simulink model "SailingYachtModel"  (R2017a)
settings: Solver=ode3  StartTime=0.0  StopTime=1800  FixedStep=0.4  RelTol=1e-3
settings Model: Creator=Administrator  LastModifiedBy=davi
settings DataIOCC: LimitDataPoints=on  SaveFormat=Array  SignalLoggingSaveFormat=ModelDataLogs
settings OptimizationCC: BlockReduction=off  BooleanDataType=off  LifeSpan=inf
settings DebuggingCC: SaveWithParameterizedLinksMsg=none  UnderspecifiedInitializationDetection=Classic  MergeDetectMultiDrivingBlocksExec=none  SignalResolutionControl=TryResolveAllWithWarning  MultiTaskDSMMsg=warning  MultiTaskCondExecSysMsg=none  StateNameClashWarn=warning  SFUnexpectedBacktrackingDiag=warning  SFNoUnconditionalDefaultTransitionDiag=warning  SFExecutionAtInitializationDiag=none
settings HardwareCC: ProdBitPerPointer=32  ProdBitPerSizeT=32  ProdBitPerPtrDiffT=32  ProdLargestAtomicFloat=None  ProdIntDivRoundTo=Undefined  ProdEndianess=Unspecified  ProdWordSize=32  ProdHWDeviceType=32-bit Generic  TargetUnknown=on
settings ModelReferenceCC: PropagateSignalLabelsOutOfModel=off
settings GRTTargetCC: TargetLangStandard=C89/C90 (ANSI)  GeneratePreprocessorConditionals=Disable all
settings ConfigComp: CovMetricSettings=dw  CovHtmlReporting=on  CovSaveCumulativeToWorkspaceVar=on  CovSaveSingleToWorkspaceVar=on  CovExternalEMLEnable=off

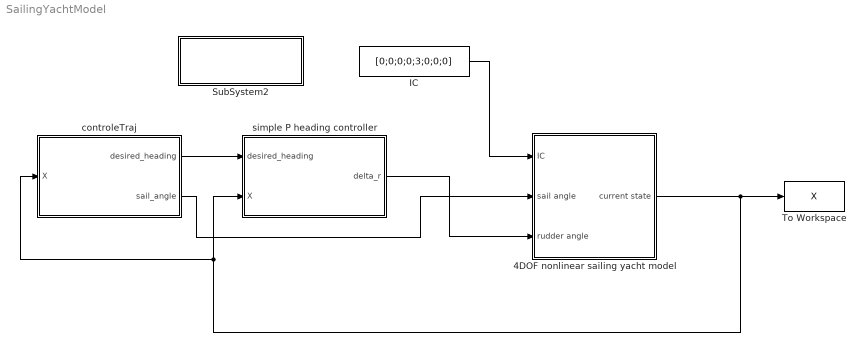
== system SailingYachtModel ==
  4DOF nonlinear sailing yacht model : Subsystem
  IC : Constant  Value=[0;0;0;0;3;0;0;0]
  SubSystem2 : Subsystem  InitFcn=|
      | global par                                                                      
      | par.dist_lateral = 0;                                                           
      | par.contador_teste = 1;                                                         
      | par.overshoot = 0;                                                              
      | par.tempopico = 0;                                                              
      | par.temposub = 0;                                                               
      | par.flagtemposub = true;                                                        
      | par.flagAcomod = false;                                                         
      | par.tempoDeAcomod = 0;                                                          
      | par.spvec = 0;                                                                  
      | par.spveccont = 1;                                                              
      | par.lastDistanciaAlvo = 0;                                                      
      | par.flag = 0;                                                                   
      | par.contador_bug = 0;                                                           
      | par.psi = 0;                                                                    
      | par.velocidade = 0;                                                             
      | par.contVel = 1;                                                                
      | par.Ianterior = 0;                                                              
      | par.distanciaAlvo = 999999999                                                   
      | w1 = [200;0];
      | w2 = [100;100];
      | w3 = [0;0];                                                                                                     
      | par.waypoints = [w1];                                                     
      | par.waypointId = 1;                                                             
      | par.nextLocation = [0;0];                                                       
      | par.waypointBId = 1;                                                            
      | par.isBordejando = false;                                                       
      | par.i = 1;                                                                      
      | par.pontos_bordejar = eye(2,1);                                                 
      | par.controle = 0;                                                               
      | par.lastlastLocation = eye(2,1);                                                
      | par.taxa_dist = 0.3;                                                            
      | par.angulo_bordejo = 40;                                                        
      | par.m = 25900;                         % (kg),mass of the vehicle               
      | par.Ixx = 133690;                                                               
      | par.Izz = 24760;                                                                
      | par.Ixz = 2180;                        % moment of inertia                      
      | par.a11 = 970;                                                                  
      | par.a22 = 17430;                                                                
      | par.a44 = 106500;                                                               
      | par.a66 = 101650;                                                               
      | par.a24 = -13160;                                                               
      | par.a26 = -6190;                                                                
      | par.a46 = 4730;                        % (kg),added mass coef.                  
      |                                                                                 
      | par.vt = 10;                           % the norm of wind velocity              
      |                                                                                 
      | par.rho_a = 1.2;                       % (kg/m^3), air density                  
      | par.As = 170;                          % (m^2), sail area                       
      | par.h0 = 0.0005;                       % (m), roughness height                  
      | par.h1 = 11.58;                        % (m), reference height                  
      | par.z_s = -11.58;                      % (m), (x,y,z) is the CoE                
      | par.xs = 0;                                                                     
      | par.ys = 0;                                                                     
      | par.zs = -11.58;                       % (m), (x,y,z) is the CoE                
      | par.Xce = 0.6;                         % (m), distance along the mast to the CoE
      | par.Xm = 0.3;                          % (m), x-coordinate of the mast          
      |                                                                                 
      | par.rho_w = 1025;                      % (kg/m^3), water density                
      | par.Ar = 1.17;                         % (m^2), rudder area                     
      | par.d_r = 1.9;                         % rudder draft                           
      | par.zeta_r = 0.8;                      % rudder efficiency                      
      | par.x_r = -8.2;                                                                 
      | par.z_r = -0.78;                       % (m), (x,y,z) is the CoE                
      | par.xr = -8.2;                                                                  
      | par.yr = 0;                                                                     
      | par.zr = -0.78;                        % (m), (x,y,z) is the CoE                
      |                                                                                 
      | par.Ak = 8.7;                          % (m^2), keel area                       
      | par.d_k = 2.49;                        % keel draft                             
      | par.zeta_k = 0.7;                      % keel efficiency                        
      | par.x_k = 0;                                                                    
      | par.z_k = -0.58;                       % (m), (x,y,z) is the CoE                
      | par.xk = 0;                                                                     
      | par.yk = 0;                                                                     
      | par.zk = -0.58;                        % (m), (x,y,z) is the CoE                
      |                                                                                 
      | par.x_h = 0;                                                                    
      | par.z_h = -1.18;                       % (m), (x,y,z) is the CoE                
      | par.xh = 0;                                                                     
      | par.yh = 0;                                                                     
      | par.zh = -1.18;                        % (m), (x,y,z) is the CoE                
      |                                                                                 
      | par.w_c = 60000;                       % (N), crew weight 20000                 
      | par.x_c = -8;                          % (m), crew position                     
      | par.y_bm = 3.6;                        % (m), yacht beam                        
      |                                                                                 
      | par.a = -5.89;                                                                  
      | par.b = 8160;                                                                   
      | par.c = 120000;                                                                 
      | par.d = 50000;
      mask Display: disp('Parameter Initialization')
  To Workspace : ToWorkspace  VariableName=X  SaveFormat=Structure With Time  SampleTime=-1
  controleTraj : Subsystem
  simple P heading controller : Subsystem
  wires:
  controleTraj/1(desired_heading) -> simple P heading controller/1(desired_heading)
  4DOF nonlinear sailing yacht model/1(current state) -> controleTraj/1(X), simple P heading controller/2(X), To Workspace/1
  IC/1 -> 4DOF nonlinear sailing yacht model/1(IC)
  controleTraj/2(sail_angle) -> 4DOF nonlinear sailing yacht model/2(sail angle)
  simple P heading controller/1(delta_r) -> 4DOF nonlinear sailing yacht model/3(rudder angle)

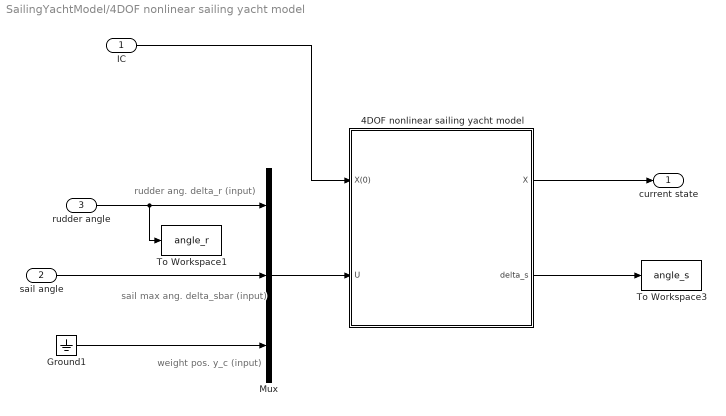
== system SailingYachtModel/4DOF nonlinear sailing yacht model ==
  note: weight pos. y_c (input)
  note: rudder ang. delta_r (input)
  note: sail max ang. delta_sbar (input)
  IC : Inport
  sail angle : Inport  Port=2
  rudder angle : Inport  Port=3
  4DOF nonlinear sailing yacht model : Subsystem
  Ground1 : Ground
  Mux : Mux  Inputs=3
  To Workspace1 : ToWorkspace  VariableName=angle_r  SaveFormat=Structure With Time  SampleTime=-1
  To Workspace3 : ToWorkspace  VariableName=angle_s  SaveFormat=Structure With Time  SampleTime=-1
  current state : Outport
  wires:
  Mux/1 -> 4DOF nonlinear sailing yacht model/2(U)
  4DOF nonlinear sailing yacht model/2(delta_s) -> To Workspace3/1
  sail angle/1 -> Mux/2
  rudder angle/1 -> To Workspace1/1, Mux/1
  4DOF nonlinear sailing yacht model/1(X) -> current state/1
  Ground1/1 -> Mux/3
  IC/1 -> 4DOF nonlinear sailing yacht model/1(X(0))

== system SailingYachtModel/SubSystem2 ==

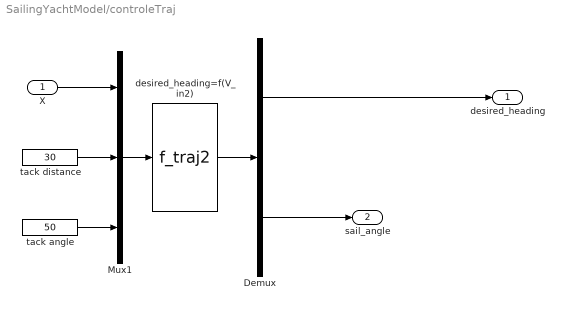
== system SailingYachtModel/controleTraj ==
  X : Inport
  Demux : Demux  Outputs=2
  Mux1 : Mux  Inputs=3
  desired_heading=f(V_in2) : MATLABFcn  MATLABFcn=f_traj2  OutputDimensions=2
  tack angle : Constant  Value=50
  tack distance : Constant  Value=30
  desired_heading : Outport
  sail_angle : Outport  Port=2
  wires:
  Demux/1 -> desired_heading/1
  Demux/2 -> sail_angle/1
  X/1 -> Mux1/1
  tack distance/1 -> Mux1/2
  tack angle/1 -> Mux1/3
  Mux1/1 -> desired_heading=f(V_in2)/1
  desired_heading=f(V_in2)/1 -> Demux/1

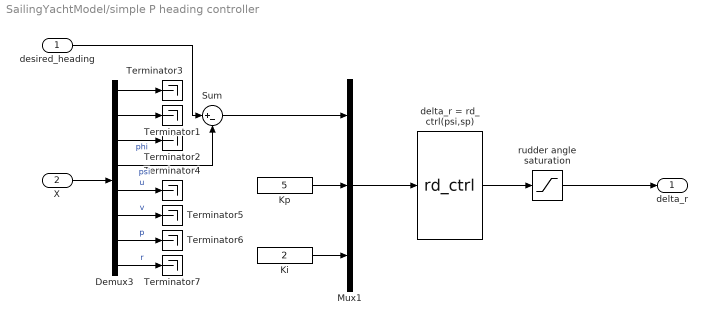
== system SailingYachtModel/simple P heading controller ==
  desired_heading : Inport
  X : Inport  Port=2
  Demux3 : Demux  Outputs=8
  Ki : Constant  Value=2
  Kp : Constant  Value=5
  Mux1 : Mux  Inputs=3
  Sum : Sum  Inputs=|+-  SaturateOnIntegerOverflow=on
  Terminator{1..7} (7 alike) : Terminator
  delta_r = rd_ctrl(psi,sp) : MATLABFcn  MATLABFcn=rd_ctrl  OutputDimensions=1
  rudder angle saturation : Saturate  UpperLimit=pi/3  LowerLimit=-pi/3  LinearizeAsGain=off
  delta_r : Outport
  wires:
  Demux3/4 -> Sum/2  "psi"
  X/1 -> Demux3/1
  Demux3/1 -> Terminator3/1
  Demux3/2 -> Terminator1/1
  Demux3/3 -> Terminator2/1  "phi"
  Demux3/5 -> Terminator4/1  "u"
  Demux3/6 -> Terminator5/1  "v"
  Demux3/7 -> Terminator6/1  "p"
  Demux3/8 -> Terminator7/1  "r"
  rudder angle saturation/1 -> delta_r/1
  delta_r = rd_ctrl(psi,sp)/1 -> rudder angle saturation/1
  desired_heading/1 -> Sum/1
  Mux1/1 -> delta_r = rd_ctrl(psi,sp)/1
  Sum/1 -> Mux1/1
  Kp/1 -> Mux1/2
  Ki/1 -> Mux1/3

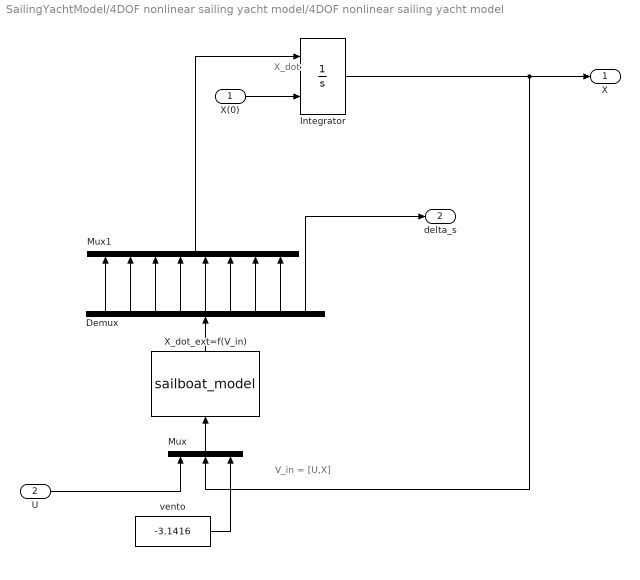
== system SailingYachtModel/4DOF nonlinear sailing yacht model/4DOF nonlinear sailing yacht model ==
  note: X_dot
  note: V_in = [U,X]
  X(0) : Inport
  U : Inport  Port=2
  Demux : Demux  Outputs=9
  Integrator : Integrator  InitialConditionSource=external  InitialCondition=[0;0;0;pi;1;0;0;0]
  Mux : Mux  Inputs=3
  Mux1 : Mux  Inputs=8
  X_dot_ext=f(V_in) : MATLABFcn  MATLABFcn=sailboat_model  OutputDimensions=9
  vento : Constant  Value=-3.1416
  X : Outport
  delta_s : Outport  Port=2
  wires:
  X(0)/1 -> Integrator/2
  Mux/1 -> X_dot_ext=f(V_in)/1
  U/1 -> Mux/1
  Integrator/1 -> X/1, Mux/2
  X_dot_ext=f(V_in)/1 -> Demux/1
  Demux/9 -> delta_s/1
  Demux/8 -> Mux1/8
  Demux/7 -> Mux1/7
  Demux/6 -> Mux1/6
  Demux/5 -> Mux1/5
  Demux/4 -> Mux1/4
  Demux/3 -> Mux1/3
  Demux/2 -> Mux1/2
  Demux/1 -> Mux1/1
  Mux1/1 -> Integrator/1
  vento/1 -> Mux/3
